simulink model "delta_kinematics"  (R2025a)
settings: Solver=ode3  StartTime=0.0  StopTime=1.2  FixedStep=0.002  RelTol=1e-3
settings Model: Creator=ACER  LastModifiedBy=ACER

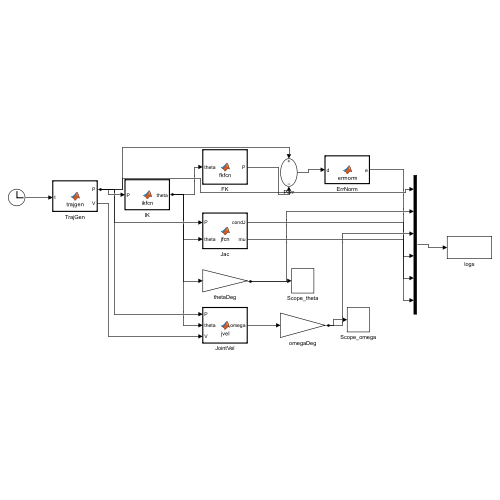
[thumbnail: Simulink's stored preview of the top-level diagram]
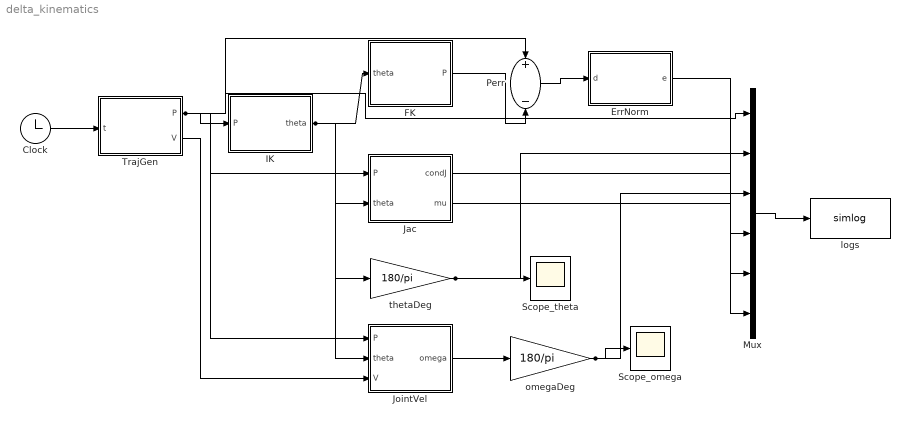
== system delta_kinematics ==
  Clock : Clock
  ErrNorm : MATLAB Function  TreatAsAtomicUnit=on
  FK : MATLAB Function  TreatAsAtomicUnit=on
  IK : MATLAB Function  TreatAsAtomicUnit=on
  Jac : MATLAB Function  TreatAsAtomicUnit=on
  JointVel : MATLAB Function  TreatAsAtomicUnit=on
  Mux : Mux  Inputs=6
  Perr : Sum  Inputs=+-
  Scope_omega : Scope
  Scope_theta : Scope
  TrajGen : MATLAB Function  TreatAsAtomicUnit=on
  logs : ToWorkspace  VariableName=simlog  SaveFormat=Timeseries  SampleTime=-1
  omegaDeg : Gain  Gain=180/pi
  thetaDeg : Gain  Gain=180/pi
  wires:
  Clock/1 -> TrajGen/1(t)
  TrajGen/1(P) -> IK/1(P), Jac/1(P), Perr/1, Mux/1, JointVel/1(P)
  TrajGen/2(V) -> JointVel/3(V)
  IK/1(theta) -> FK/1(theta), Jac/2(theta), thetaDeg/1, JointVel/2(theta)
  FK/1(P) -> Perr/2
  Perr/1 -> ErrNorm/1(d)
  thetaDeg/1 -> Mux/2, Scope_theta/1
  JointVel/1(omega) -> omegaDeg/1
  omegaDeg/1 -> Mux/3, Scope_omega/1
  Jac/1(condJ) -> Mux/4
  Jac/2(mu) -> Mux/5
  ErrNorm/1(e) -> Mux/6
  Mux/1 -> logs/1

== matlab function delta_kinematics/TrajGen ==
  data: t input; P output; V output
function [P, V] = trajgen(t)
%#codegen
W = [ 300 0 -1000; 300 0 -820; -300 0 -820; -300 0 -1000];
Tseg = [0.30 0.60 0.30];
Tend = sum(Tseg);
tt = mod(t, Tend);
if tt <= Tseg(1)
    k = 1; t0 = 0;
elseif tt <= Tseg(1)+Tseg(2)
    k = 2; t0 = Tseg(1);
else
    k = 3; t0 = Tseg(1)+Tseg(2);
end
Tk = Tseg(k);
s = (tt - t0)/Tk;
if s<0, s=0; end
if s>1, s=1; end
ss = 10*s^3 - 15*s^4 + 6*s^5;
ssd = (30*s^2 - 60*s^3 + 30*s^4)/Tk;
A = W(k,:); B = W(k+1,:);
Pv = A + ss*(B - A);
Vv = ssd*(B - A);
P = Pv(:); V = Vv(:);
end

== matlab function delta_kinematics/FK ==
  data: theta input; P output
function P = fkfcn(theta)
%#codegen
R=347.0; r=120.6; L1=407.5; L2=1000.0;
phi=[-pi/2, pi/6, 5*pi/6];
C=zeros(3,3);
for i=1:3
  c=cos(phi(i)); s=sin(phi(i)); ct=cos(theta(i)); st=sin(theta(i));
  Ex=R*c+L1*ct*c; Ey=R*s+L1*ct*s; Ez=-L1*st;
  C(i,:)=[Ex-r*c, Ey-r*s, Ez];
end
c1=C(1,:); c2=C(2,:); c3=C(3,:);
A=2*[c2-c1; c3-c1];
bb=[sum(c2.^2)-sum(c1.^2); sum(c3.^2)-sum(c1.^2)];
d=cross(A(1,:),A(2,:));
P=[NaN;NaN;NaN];
if norm(d)<1e-9, return; end
M=A*A';
P0=(A'*(M\bb))';
aa=dot(d,d); bq=2*dot(d,P0-c1); cq=dot(P0-c1,P0-c1)-L2^2;
disc=bq^2-4*aa*cq;
if disc<0
  if disc>-1e-6, disc=0; else, return; end
end
t1=(-bq+sqrt(disc))/(2*aa); t2=(-bq-sqrt(disc))/(2*aa);
Pa=P0+t1*d; Pb=P0+t2*d;
if Pa(3)<=Pb(3), Pv=Pa; else, Pv=Pb; end
P=Pv(:);
end

== matlab function delta_kinematics/Jac ==
  data: P input; condJ output; theta input; mu output
function [condJ, mu] = jfcn(P, theta)
%#codegen
R=347.0; r=120.6; L1=407.5;
phi=[-pi/2, pi/6, 5*pi/6];
A=zeros(3,3); bd=zeros(3,1); mus=zeros(3,1);
for i=1:3
  c=cos(phi(i)); s=sin(phi(i)); ct=cos(theta(i)); st=sin(theta(i));
  Bi=[R*c; R*s; 0];
  Ei=[R*c+L1*ct*c; R*s+L1*ct*s; -L1*st];
  Pi=[P(1)+r*c; P(2)+r*s; P(3)];
  Li=Ei-Pi;
  A(i,:)=Li';
  vhat=[-st*c; -st*s; -ct];
  bd(i)=L1*(Li'*vhat);
  bicep=Ei-Bi;
  cosb=(Li'*bicep)/(norm(Li)*norm(bicep));
  mus(i)=acos(max(-1,min(1,abs(cosb))))*180/pi;
end
B=diag(bd);
if abs(det(A))<1e-9
  condJ=1e6;
else
  Jf=A\B;
  condJ=cond(Jf);
end
mu=min(mus);
end

== matlab function delta_kinematics/ErrNorm ==
  data: d input; e output
function e = errnorm(d)
%#codegen
e = norm(d);
end

== matlab function delta_kinematics/JointVel ==
  data: P input; omega output; theta input; V input
function omega = jvel(P, theta, V)
%#codegen
R=347.0; r=120.6; L1=407.5;
phi=[-pi/2, pi/6, 5*pi/6];
omega=zeros(3,1);
for i=1:3
  c=cos(phi(i)); s=sin(phi(i)); ct=cos(theta(i)); st=sin(theta(i));
  Ei=[R*c+L1*ct*c; R*s+L1*ct*s; -L1*st];
  Pi=[P(1)+r*c; P(2)+r*s; P(3)];
  Li=Ei-Pi;
  vhat=[-st*c; -st*s; -ct];
  bden=L1*(Li'*vhat);
  if abs(bden)<1e-9
    omega(i)=0;
  else
    omega(i)=(Li'*V)/bden;
  end
end
end

== matlab function delta_kinematics/IK ==
  data: P input; theta output
function theta = ikfcn(P)
%#codegen
R=347.0; r=120.6; Rr=R-r; L1=407.5; L2=1000.0;
phi=[-pi/2, pi/6, 5*pi/6];
th_min=-pi/4; th_max=100*pi/180;
theta=zeros(3,1);
for i=1:3
  c=cos(phi(i)); s=sin(phi(i));
  u=(P(1)*c+P(2)*s)-Rr;
  w=-P(1)*s+P(2)*c;
  z=P(3);
  E=2*L1*z; F=-2*L1*u; G=L1^2+u^2+w^2+z^2-L2^2;
  rho=hypot(E,F);
  if rho<1e-12 || abs(G)>rho+1e-6
    theta(i)=NaN; continue;
  end
  psi=atan2(F,E);
  as=max(-1,min(1,-G/rho));
  b=asin(as);
  c1=atan2(sin(b-psi),cos(b-psi));
  c2=atan2(sin(pi-b-psi),cos(pi-b-psi));
  in1=(c1>=th_min && c1<=th_max);
  in2=(c2>=th_min && c2<=th_max);
  if in1 && in2
    theta(i)=min(c1,c2);
  elseif in1
    theta(i)=c1;
  elseif in2
    theta(i)=c2;
  else
    theta(i)=c1;
  end
end
end
